simulink model "Template"  (R2022a)
settings: Solver=FixedStepAuto  StartTime=0.0  StopTime=inf  RelTol=1e-3  EnableMultiTasking=on
libraries: Lab_Blocks_4M25 x3
settings Model: Creator=ronan  LastModifiedBy=ronan
settings OptimizationCC: EnhancedBackFolding=on  PassReuseOutputArgsAs=Individual arguments  ZeroExternalMemoryAtStartup=off  ZeroInternalMemoryAtStartup=off  MaxStackSize=64  OptimizeBlockOrder=speed  DifferentSizesBufferReuse=on  OptimizationCustomize=off  EfficientTunableParamExpr=on
settings DebuggingCC: ParameterTunabilityLossMsg=error
settings HardwareCC: ProdBitPerPointer=32  ProdBitPerSizeT=32  ProdBitPerPtrDiffT=32  ProdLargestAtomicInteger=Long  ProdLargestAtomicFloat=Double  ProdWordSize=32  ProdHWDeviceType=ARM Compatible->ARM Cortex
settings SFSimCC: MATLABDynamicMemAlloc=off
settings RTWCC: SystemTargetFile=ert.tlc  HardwareBoard=VEX V5 Robot Brain  TLCOptions="-aInlineSetEventsForThisBaseRateFcn=TLC_FALSE -aSuppressMultiTaskScheduler=TLC_FALSE  -aRateBasedStepFcn=0"  TemplateMakefile=ert_default_tmf  Toolchain=GNU Tools for ARM Embedded Processors
settings CodeAppCC: ForceParamTrailComments=on  IgnoreCustomStorageClasses=off  OperatorAnnotations=on  SimulinkDataObjDesc=on  SFDataObjDesc=on  InsertBlockDesc=on
settings ERTTargetCC: SupportContinuousTime=on  ExtModeTransport=3  ExtModeStaticAlloc=on  ExtModeStaticAllocSize=2048  ExtModeMexFile=ext_xcp  ExtModeIntrfLevel=Level2 - Open

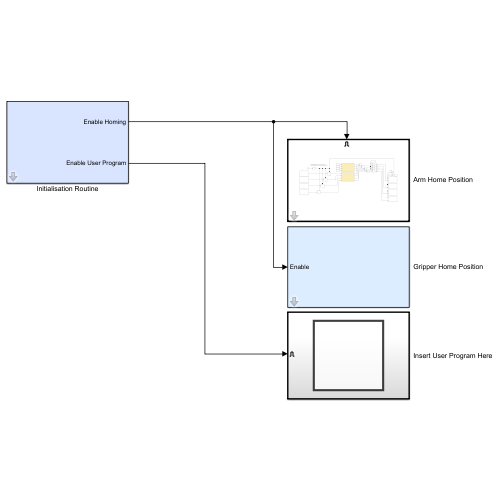
[thumbnail: Simulink's stored preview of the top-level diagram]
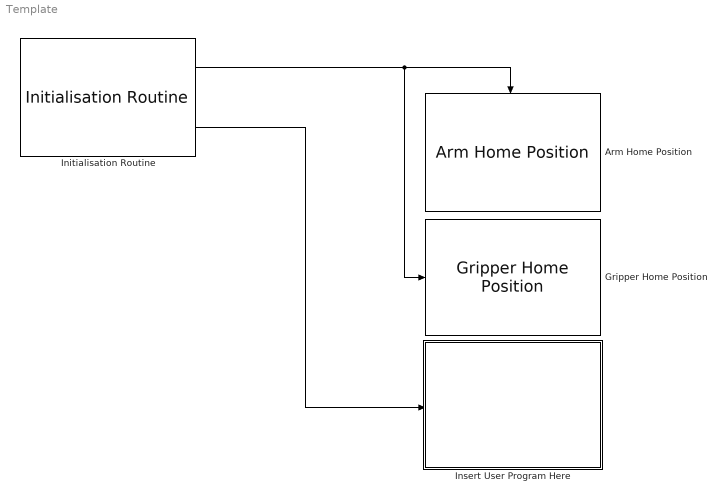
== system Template ==
  Arm Home Position : Lab_Blocks_4M25/Derived Blocks/Arm Home Position  home_A=1900  home_B=1650  home_C=1235  home_D=420  SampleTime=0.01
      settings: SourceProductName=4M25 Lab Blocks
  Gripper Home Position : Lab_Blocks_4M25/Core Blocks/Gripper Home Position  SampleTime=0.01  motorPort_right=6  motorPort_left=5
      settings: SourceProductName=4M25 Lab Blocks
  Initialisation Routine : Lab_Blocks_4M25/Core Blocks/Initialisation Routine
      settings: SourceProductName=4M25 Lab Blocks
  Insert User Program Here : Subsystem  TreatAsAtomicUnit=on
  wires:
  Initialisation Routine/1 -> Gripper Home Position/1, Arm Home Position/Enable
  Initialisation Routine/2 -> Insert User Program Here/Enable

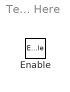
== system Template/Insert User Program Here ==
  Enable : EnablePort
